simulink library "libraryMatlab"  (R2020b)
settings: Solver=VariableStepAuto  StartTime=0.0  StopTime=10.0  RelTol=1e-3
values from neighbouring files (symbols this model uses):
  a = 7271    [linearControlTuning.m]
  data = struct()    [config.m]
undefined symbols (not defined in the file or in its folder): SRP
libraries: simulink x2
settings Model: Creator=pacif  LastModifiedBy=pacif

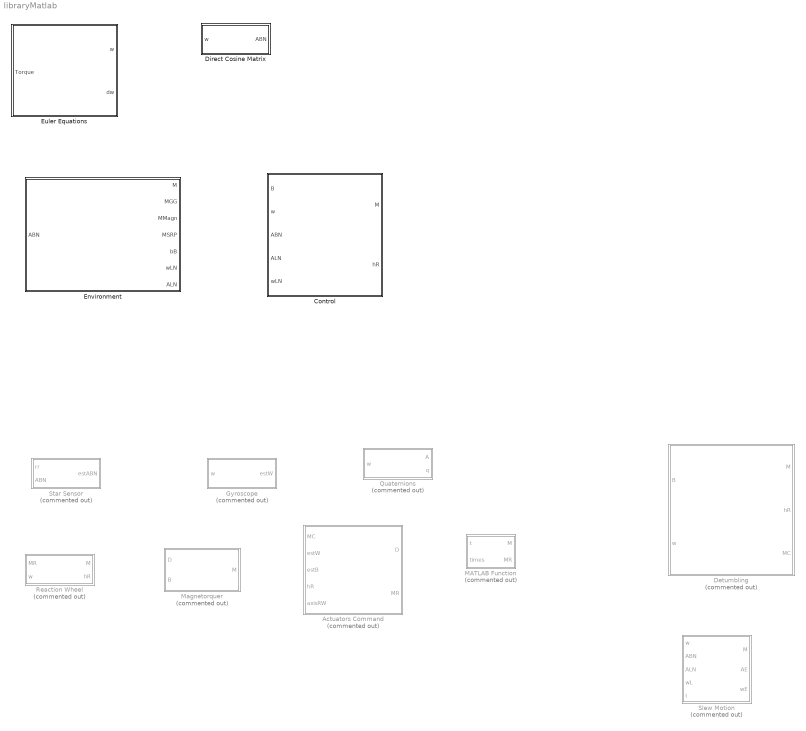
== system libraryMatlab ==
  Actuators Command : MATLAB Function  Commented=on  TreatAsAtomicUnit=on
  Control : Subsystem
  Detumbling : Subsystem  Commented=on
  Direct Cosine Matrix : Subsystem
  Environment : Subsystem
  Euler Equations : Subsystem
  Gyroscope : Subsystem  Commented=on
  MATLAB Function : MATLAB Function  Commented=on  TreatAsAtomicUnit=on
  Magnetorquer : MATLAB Function  Commented=on  TreatAsAtomicUnit=on
  Quaternions : Subsystem  Commented=on
  Reaction Wheel : Subsystem  Commented=on
  Slew Motion : MATLAB Function  Commented=on  TreatAsAtomicUnit=on
  Star Sensor : Subsystem  Commented=on

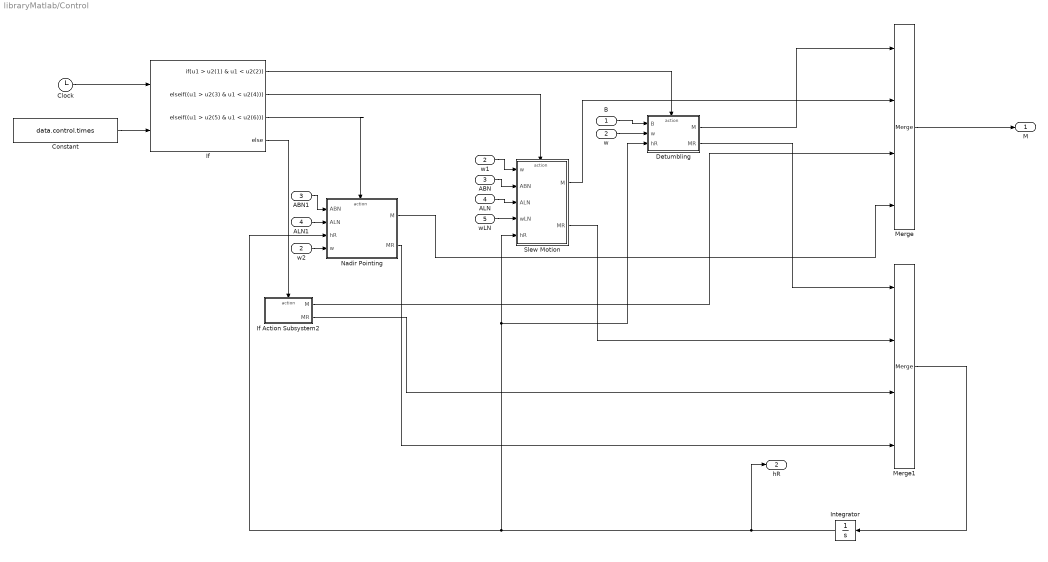
== system libraryMatlab/Control ==
  B : Inport
  w : Inport  Port=2
  ABN : Inport  Port=3
  ALN : Inport  Port=4
  wLN : Inport  Port=5
  ABN1 : InportShadow  Port=3
  ALN1 : InportShadow  Port=4
  Clock : Clock
  Constant : Constant  Value=data.control.times
  Detumbling : Subsystem  TreatAsAtomicUnit=on
  If : If  NumInputs=2  IfExpression=u1 > u2(1) & u1 < u2(2)  ElseIfExpressions=(u1 > u2(3) & u1 < u2(4)),(u1 > u2(5) & u1 < u2(6))
  If Action Subsystem2 : Subsystem  AncestorBlock=libraryMatlab/Control/Detumbling/If Action Subsystem2  TreatAsAtomicUnit=on
  Integrator : Integrator  InitialCondition=data.reactionWheel.h0
  Merge : Merge  Inputs=4
  Merge1 : Merge  Inputs=4
  Nadir Pointing : Subsystem  TreatAsAtomicUnit=on
  Slew Motion : Subsystem  TreatAsAtomicUnit=on
  w1 : InportShadow  Port=2
  w2 : InportShadow  Port=2
  M : Outport
  hR : Outport  Port=2
  wires:
  If/4 -> If Action Subsystem2/Action
  If/2 -> Slew Motion/Action
  If/1 -> Detumbling/Action
  Detumbling/1(M) -> Merge/1
  Slew Motion/1(M) -> Merge/2
  If Action Subsystem2/1(M) -> Merge/3
  Clock/1 -> If/1
  Constant/1 -> If/2
  B/1 -> Detumbling/1(B)
  w/1 -> Detumbling/2(w)
  w1/1 -> Slew Motion/1(w)
  ABN/1 -> Slew Motion/2(ABN)
  ALN/1 -> Slew Motion/3(ALN)
  wLN/1 -> Slew Motion/4(wLN)
  Merge/1 -> M/1
  Integrator/1 -> Nadir Pointing/3(hR), Detumbling/3(hR), Slew Motion/5(hR), hR/1
  Merge1/1 -> Integrator/1
  Detumbling/2(MR) -> Merge1/1
  Slew Motion/2(MR) -> Merge1/2
  If Action Subsystem2/2(MR) -> Merge1/3
  If/3 -> Nadir Pointing/Action
  Nadir Pointing/1(M) -> Merge/4
  ABN1/1 -> Nadir Pointing/1(ABN)
  ALN1/1 -> Nadir Pointing/2(ALN)
  Nadir Pointing/2(MR) -> Merge1/4
  w2/1 -> Nadir Pointing/4(w)

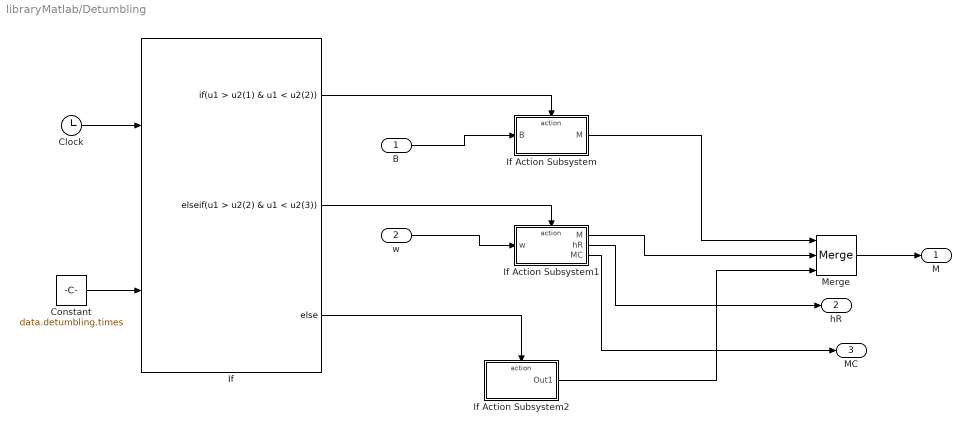
== system libraryMatlab/Detumbling ==
  B : Inport
  w : Inport  Port=2
  Clock : Clock
  Constant : Constant  Value=data.detumbling.times
  If : If  NumInputs=2  IfExpression=u1 > u2(1) & u1 < u2(2)  ElseIfExpressions=u1 > u2(2) & u1 < u2(3)
  If Action Subsystem : Subsystem  TreatAsAtomicUnit=on
  If Action Subsystem1 : Subsystem  TreatAsAtomicUnit=on
  If Action Subsystem2 : Subsystem  TreatAsAtomicUnit=on
  Merge : Merge  Inputs=3
  M : Outport
  hR : Outport  Port=2
  MC : Outport  Port=3
  wires:
  Clock/1 -> If/1
  If/1 -> If Action Subsystem/Action
  If/2 -> If Action Subsystem1/Action
  If/3 -> If Action Subsystem2/Action
  Merge/1 -> M/1
  If Action Subsystem2/1(Out1) -> Merge/3
  If Action Subsystem1/1(M) -> Merge/2
  If Action Subsystem/1(M) -> Merge/1
  B/1 -> If Action Subsystem/1(B)
  w/1 -> If Action Subsystem1/1(w)
  Constant/1 -> If/2
  If Action Subsystem1/2(hR) -> hR/1
  If Action Subsystem1/3(MC) -> MC/1

== system libraryMatlab/Direct Cosine Matrix ==
  w : Inport
  Integrator : Integrator  InitialCondition=data.ic.dcm
  MATLAB Function : MATLAB Function  TreatAsAtomicUnit=on
  MATLAB Function1 : MATLAB Function  TreatAsAtomicUnit=on
  ABN : Outport
  wires:
  w/1 -> MATLAB Function/2(w)
  MATLAB Function/1(dA) -> Integrator/1
  Integrator/1 -> MATLAB Function1/1(A0)
  MATLAB Function1/1(A) -> ABN/1, MATLAB Function/1(A)

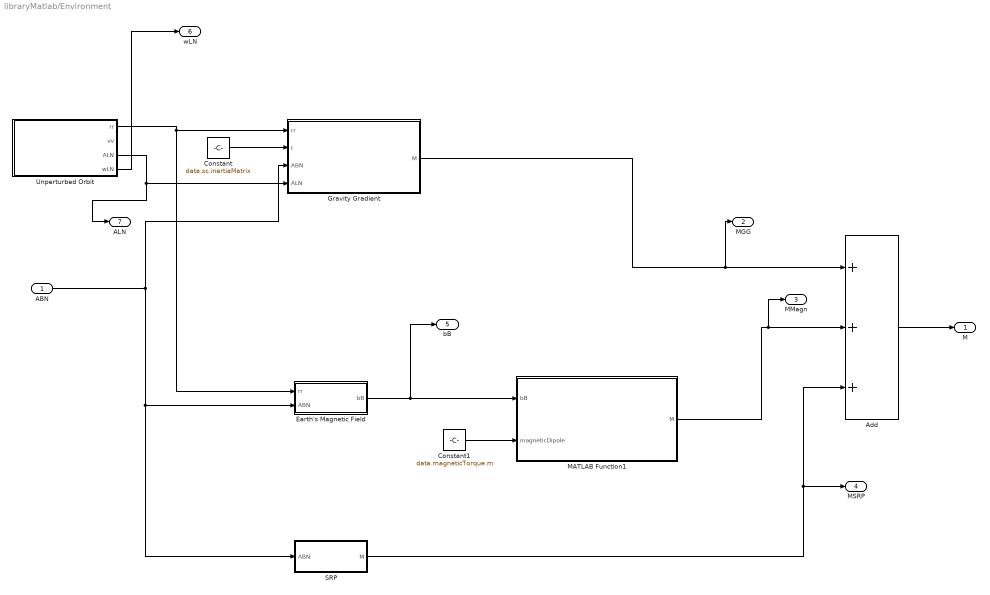
== system libraryMatlab/Environment ==
  ABN : Inport
  Add : Sum  Inputs=+++
  Constant : Constant  Value=data.sc.inertiaMatrix
  Constant1 : Constant  Value=data.magneticTorque.m
  Earth's Magnetic Field : Subsystem
  Gravity Gradient : MATLAB Function  TreatAsAtomicUnit=on
  MATLAB Function1 : MATLAB Function  TreatAsAtomicUnit=on
  SRP : Subsystem  AncestorBlock=a/SRP
  Unperturbed Orbit : Subsystem
  M : Outport
  MGG : Outport  Port=2
  MMagn : Outport  Port=3
  MSRP : Outport  Port=4
  bB : Outport  Port=5
  wLN : Outport  Port=6
  ALN : Outport  Port=7
  wires:
  Unperturbed Orbit/1(rr) -> Earth's Magnetic Field/1(rr), Gravity Gradient/1(rr)
  Unperturbed Orbit/3(ALN) -> ALN/1, Gravity Gradient/4(ALN)
  Constant/1 -> Gravity Gradient/2(I)
  Constant1/1 -> MATLAB Function1/2(magneticDipole)
  ABN/1 -> Gravity Gradient/3(ABN), Earth's Magnetic Field/2(ABN), SRP/1(ABN)
  MATLAB Function1/1(M) -> Add/2, MMagn/1
  Earth's Magnetic Field/1(bB) -> bB/1, MATLAB Function1/1(bB)
  Gravity Gradient/1(M) -> MGG/1, Add/1
  SRP/1(M) -> MSRP/1, Add/3
  Add/1 -> M/1
  Unperturbed Orbit/4(wLN) -> wLN/1

== system libraryMatlab/Euler Equations ==
  Torque : Inport
  Constant : Constant  Value=data.sc.inertiaMatrix
  Integrator : Integrator  InitialCondition=data.ic.w
  MATLAB Function : MATLAB Function  TreatAsAtomicUnit=on
  w : Outport
  dw : Outport  Port=2
  wires:
  Constant/1 -> MATLAB Function/3(I)
  Integrator/1 -> w/1, MATLAB Function/1(w)
  Torque/1 -> MATLAB Function/2(M)
  MATLAB Function/1(dw) -> dw/1, Integrator/1

== system libraryMatlab/Gyroscope ==
  w : Inport
  Add : Sum  Inputs=+++
  Band-Limited White Noise : simulink/Sources/Band-Limited White Noise  Cov=[1; 1; 1]  Ts=data.gyroscope.sampleTime  seed=[23341]
  Band-Limited White Noise1 : simulink/Sources/Band-Limited White Noise  Cov=[1; 1; 1]  Ts=data.gyroscope.sampleTime  seed=[23341]
  Gain : Gain  Gain=data.gyroscope.sigmaN
  Gain1 : Gain  Gain=data.gyroscope.sigmaB
  Integrator : Integrator  InitialCondition=[0;0;0]
  estW : Outport
  wires:
  Band-Limited White Noise/1 -> Gain/1
  Gain/1 -> Add/2  "n"
  Gain1/1 -> Integrator/1  "bDot"
  Integrator/1 -> Add/3  "b"
  w/1 -> Add/1
  Add/1 -> estW/1
  Band-Limited White Noise1/1 -> Gain1/1

== system libraryMatlab/Quaternions ==
  w : Inport
  Integrator : Integrator  InitialCondition=data.ic.quaternions
  MATLAB Function : MATLAB Function  TreatAsAtomicUnit=on
  MATLAB Function1 : MATLAB Function  TreatAsAtomicUnit=on
  MATLAB Function2 : MATLAB Function  TreatAsAtomicUnit=on
  A : Outport
  q : Outport  Port=2
  wires:
  w/1 -> MATLAB Function/2(w)
  MATLAB Function/1(dq) -> Integrator/1
  Integrator/1 -> MATLAB Function2/1(q0)
  MATLAB Function2/1(q) -> MATLAB Function/1(q), q/1, MATLAB Function1/1(q)
  MATLAB Function1/1(A) -> A/1

== system libraryMatlab/Reaction Wheel ==
  MR : Inport
  w : Inport  Port=2
  Constant : Constant  Value=data.reactionWheel.axes
  Integrator : Integrator
  MATLAB Function : MATLAB Function  TreatAsAtomicUnit=on
  M : Outport
  hR : Outport  Port=2
  wires:
  MR/1 -> MATLAB Function/2(MR), Integrator/1
  Integrator/1 -> hR/1, MATLAB Function/1(hR)  "hR"
  Constant/1 -> MATLAB Function/4(axesRW)
  w/1 -> MATLAB Function/3(w)
  MATLAB Function/1(M) -> M/1

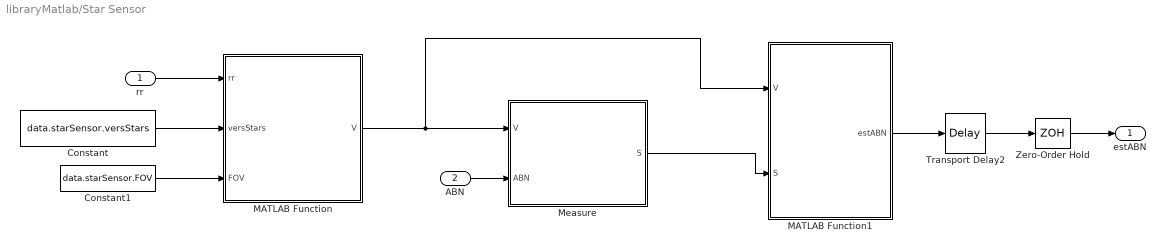
== system libraryMatlab/Star Sensor ==
  rr : Inport
  ABN : Inport  Port=2
  Constant : Constant  Value=data.starSensor.versStars
  Constant1 : Constant  Value=data.starSensor.FOV
  MATLAB Function : MATLAB Function  TreatAsAtomicUnit=on
  MATLAB Function1 : MATLAB Function  TreatAsAtomicUnit=on
  Measure : Subsystem
  Transport Delay2 : TransportDelay  DelayTime=data.starSensor.sampleTime
  Zero-Order Hold : ZeroOrderHold  SampleTime=data.starSensor.sampleTime
  estABN : Outport
  wires:
  Constant/1 -> MATLAB Function/2(versStars)
  Constant1/1 -> MATLAB Function/3(FOV)
  Measure/1(S) -> MATLAB Function1/2(S)
  ABN/1 -> Measure/2(ABN)
  Zero-Order Hold/1 -> estABN/1
  rr/1 -> MATLAB Function/1(rr)
  MATLAB Function/1(V) -> MATLAB Function1/1(V), Measure/1(V)
  MATLAB Function1/1(estABN) -> Transport Delay2/1
  Transport Delay2/1 -> Zero-Order Hold/1

== system libraryMatlab/Control/Detumbling ==
  B : Inport
  w : Inport  Port=2
  hR : Inport  Port=3
  Action Port : ActionPort  ActionPortLabel=if(u1 > u2(1) & u1 < u2(2))
  Detumbling : Subsystem  AncestorBlock=libraryMatlab/Detumbling
  M : Outport
  MR : Outport  Port=2
  wires:
  Detumbling/1(M) -> M/1
  B/1 -> Detumbling/1(B)
  w/1 -> Detumbling/2(w)
  Detumbling/2(MR) -> MR/1
  hR/1 -> Detumbling/3(hR)

== system libraryMatlab/Control/If Action Subsystem2 ==
  Action Port : ActionPort  ActionPortLabel=else
  Constant : Constant  Value=[0;0;0]
  Constant1 : Constant  Value=0*data.reactionWheel.h0  VectorParams1D=off
  M : Outport
  MR : Outport  Port=2
  wires:
  Constant/1 -> M/1
  Constant1/1 -> MR/1

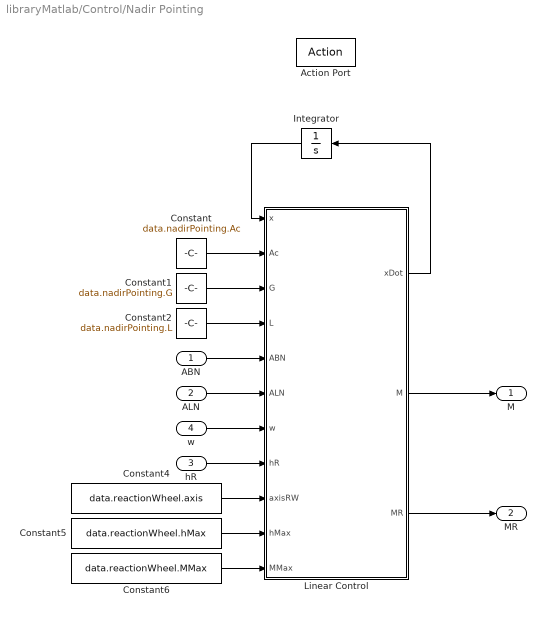
== system libraryMatlab/Control/Nadir Pointing ==
  ABN : Inport
  ALN : Inport  Port=2
  hR : Inport  Port=3
  w : Inport  Port=4
  Action Port : ActionPort  ActionPortLabel=elseif((u1 > u2(5) & u1 < u2(6)))
  Constant : Constant  Value=data.nadirPointing.Ac
  Constant1 : Constant  Value=data.nadirPointing.G
  Constant2 : Constant  Value=data.nadirPointing.L
  Constant4 : Constant  Value=data.reactionWheel.axis
  Constant5 : Constant  Value=data.reactionWheel.hMax
  Constant6 : Constant  Value=data.reactionWheel.MMax
  Integrator : Integrator  InitialCondition=zeros(6,1)
  Linear Control : MATLAB Function  TreatAsAtomicUnit=on
  M : Outport
  MR : Outport  Port=2
  wires:
  ALN/1 -> Linear Control/6(ALN)
  ABN/1 -> Linear Control/5(ABN)
  Linear Control/2(M) -> M/1
  Linear Control/1(xDot) -> Integrator/1
  Integrator/1 -> Linear Control/1(x)
  Constant/1 -> Linear Control/2(Ac)
  Constant2/1 -> Linear Control/4(L)
  Constant1/1 -> Linear Control/3(G)
  Constant4/1 -> Linear Control/9(axisRW)
  Constant5/1 -> Linear Control/10(hMax)
  Constant6/1 -> Linear Control/11(MMax)
  hR/1 -> Linear Control/8(hR)
  Linear Control/3(MR) -> MR/1
  w/1 -> Linear Control/7(w)

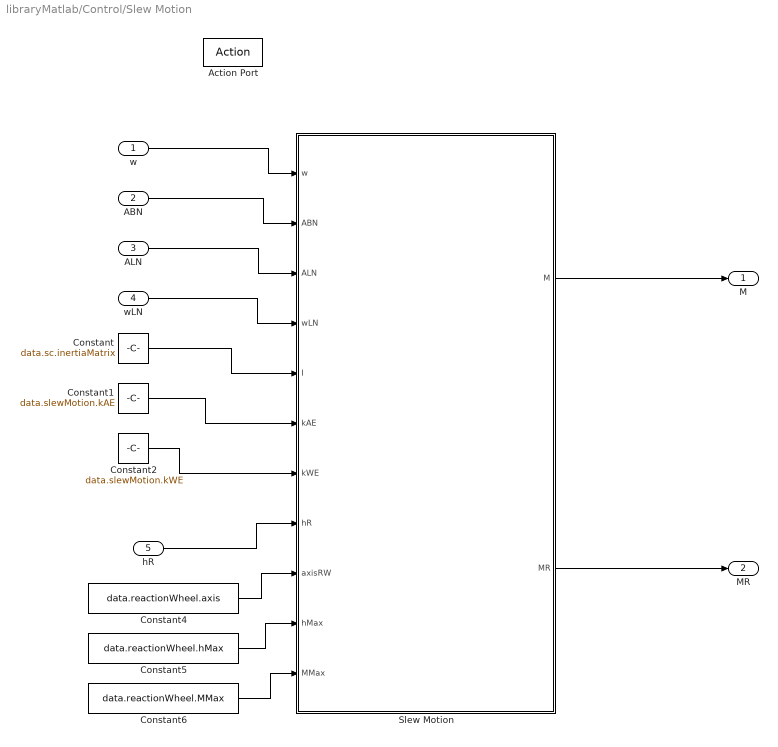
== system libraryMatlab/Control/Slew Motion ==
  w : Inport
  ABN : Inport  Port=2
  ALN : Inport  Port=3
  wLN : Inport  Port=4
  hR : Inport  Port=5
  Action Port : ActionPort  ActionPortLabel=elseif(u1 > u2(3) & u1 < u2(4))
  Constant : Constant  Value=data.sc.inertiaMatrix
  Constant1 : Constant  Value=data.slewMotion.kAE
  Constant2 : Constant  Value=data.slewMotion.kWE
  Constant4 : Constant  Value=data.reactionWheel.axis
  Constant5 : Constant  Value=data.reactionWheel.hMax
  Constant6 : Constant  Value=data.reactionWheel.MMax
  Slew Motion : MATLAB Function  TreatAsAtomicUnit=on
  M : Outport
  MR : Outport  Port=2
  wires:
  Slew Motion/1(M) -> M/1
  w/1 -> Slew Motion/1(w)
  ABN/1 -> Slew Motion/2(ABN)
  ALN/1 -> Slew Motion/3(ALN)
  wLN/1 -> Slew Motion/4(wLN)
  Constant/1 -> Slew Motion/5(I)
  Constant1/1 -> Slew Motion/6(kAE)
  Constant2/1 -> Slew Motion/7(kWE)
  Slew Motion/2(MR) -> MR/1
  hR/1 -> Slew Motion/8(hR)
  Constant5/1 -> Slew Motion/10(hMax)
  Constant4/1 -> Slew Motion/9(axisRW)
  Constant6/1 -> Slew Motion/11(MMax)

== system libraryMatlab/Detumbling/If Action Subsystem ==
  B : Inport
  Action Port : ActionPort  ActionPortLabel=if(u1 > u2(1) & u1 < u2(2))
  Constant : Constant  Value=data.magnetorquer.m0
  Derivative : Derivative  CoefficientInTFapproximation=0
  Spin Rate Damping : MATLAB Function  TreatAsAtomicUnit=on
  M : Outport
  wires:
  Constant/1 -> Spin Rate Damping/1(m0)
  B/1 -> Spin Rate Damping/2(B), Derivative/1
  Spin Rate Damping/1(M) -> M/1
  Derivative/1 -> Spin Rate Damping/3(BDot)

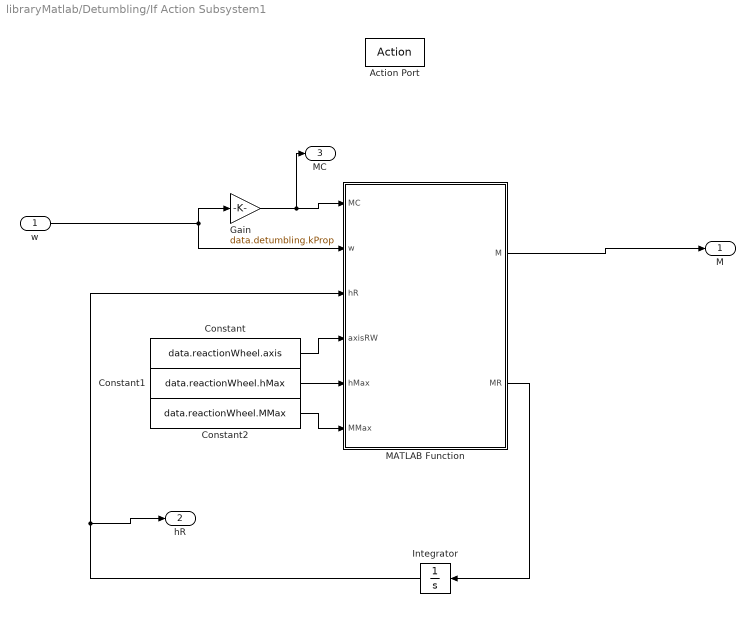
== system libraryMatlab/Detumbling/If Action Subsystem1 ==
  w : Inport
  Action Port : ActionPort  ActionPortLabel=elseif(u1 > u2(2) & u1 < u2(3))
  Constant : Constant  Value=data.reactionWheel.axis
  Constant1 : Constant  Value=data.reactionWheel.hMax
  Constant2 : Constant  Value=data.reactionWheel.MMax
  Gain : Gain  Gain=data.detumbling.kProp
  Integrator : Integrator  InitialCondition=data.reactionWheel.h0
  MATLAB Function : MATLAB Function  TreatAsAtomicUnit=on
  M : Outport
  hR : Outport  Port=2
  MC : Outport  Port=3
  wires:
  w/1 -> Gain/1, MATLAB Function/2(w)
  Gain/1 -> MC/1, MATLAB Function/1(MC)
  MATLAB Function/2(MR) -> Integrator/1
  MATLAB Function/1(M) -> M/1
  Constant/1 -> MATLAB Function/4(axisRW)
  Constant1/1 -> MATLAB Function/5(hMax)
  Constant2/1 -> MATLAB Function/6(MMax)
  Integrator/1 -> hR/1, MATLAB Function/3(hR)

== system libraryMatlab/Detumbling/If Action Subsystem2 ==
  Action Port : ActionPort  ActionPortLabel=else
  Constant : Constant  Value=[0;0;0]
  Out1 : Outport
  wires:
  Constant/1 -> Out1/1

== system libraryMatlab/Environment/Earth's Magnetic Field ==
  rr : Inport
  ABN : Inport  Port=2
  Clock : Clock
  Earth's Magnetic Field : MATLAB Function  TreatAsAtomicUnit=on
  bB : Outport
  wires:
  Earth's Magnetic Field/1(bB) -> bB/1
  rr/1 -> Earth's Magnetic Field/2(rr)
  ABN/1 -> Earth's Magnetic Field/3(ABN)
  Clock/1 -> Earth's Magnetic Field/1(t)

== system libraryMatlab/Environment/SRP ==
  ABN : Inport
  Clock : Clock
  Constant : Constant  Value=data.SRP.rhoS
  Constant1 : Constant  Value=data.SRP.rhoD
  Constant2 : Constant  Value=data.SRP.NBMat
  Constant3 : Constant  Value=data.SRP.rSurf
  Constant4 : Constant  Value=data.SRP.aSurf
  MATLAB Function : MATLAB Function  TreatAsAtomicUnit=on
  M : Outport
  wires:
  Constant4/1 -> MATLAB Function/7(aSurf)
  Constant3/1 -> MATLAB Function/6(rSurf)
  Constant2/1 -> MATLAB Function/5(NBMat)
  Constant1/1 -> MATLAB Function/4(rhoD)
  Constant/1 -> MATLAB Function/3(rhoS)
  Clock/1 -> MATLAB Function/1(t)
  MATLAB Function/1(M) -> M/1
  ABN/1 -> MATLAB Function/2(ABN)

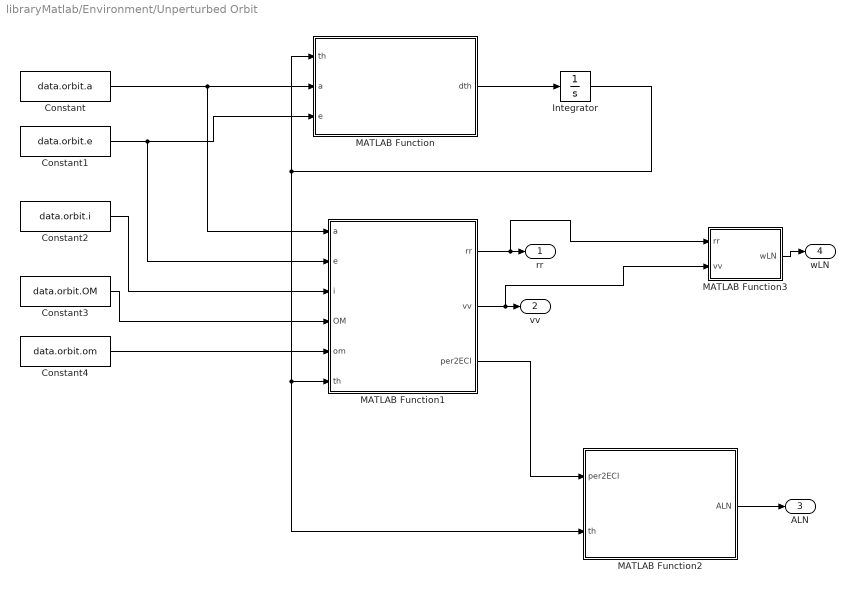
== system libraryMatlab/Environment/Unperturbed Orbit ==
  Constant : Constant  Value=data.orbit.a
  Constant1 : Constant  Value=data.orbit.e
  Constant2 : Constant  Value=data.orbit.i
  Constant3 : Constant  Value=data.orbit.OM
  Constant4 : Constant  Value=data.orbit.om
  Integrator : Integrator  InitialCondition=data.ic.th
  MATLAB Function : MATLAB Function  TreatAsAtomicUnit=on
  MATLAB Function1 : MATLAB Function  TreatAsAtomicUnit=on
  MATLAB Function2 : MATLAB Function  TreatAsAtomicUnit=on
  MATLAB Function3 : MATLAB Function  TreatAsAtomicUnit=on
  rr : Outport
  vv : Outport  Port=2
  ALN : Outport  Port=3
  wLN : Outport  Port=4
  wires:
  Constant/1 -> MATLAB Function1/1(a), MATLAB Function/2(a)
  Constant1/1 -> MATLAB Function1/2(e), MATLAB Function/3(e)
  MATLAB Function/1(dth) -> Integrator/1
  Integrator/1 -> MATLAB Function2/2(th), MATLAB Function1/6(th), MATLAB Function/1(th)
  Constant2/1 -> MATLAB Function1/3(i)
  Constant3/1 -> MATLAB Function1/4(OM)
  Constant4/1 -> MATLAB Function1/5(om)
  MATLAB Function1/1(rr) -> MATLAB Function3/1(rr), rr/1
  MATLAB Function1/2(vv) -> MATLAB Function3/2(vv), vv/1
  MATLAB Function1/3(per2ECI) -> MATLAB Function2/1(per2ECI)
  MATLAB Function2/1(ALN) -> ALN/1
  MATLAB Function3/1(wLN) -> wLN/1

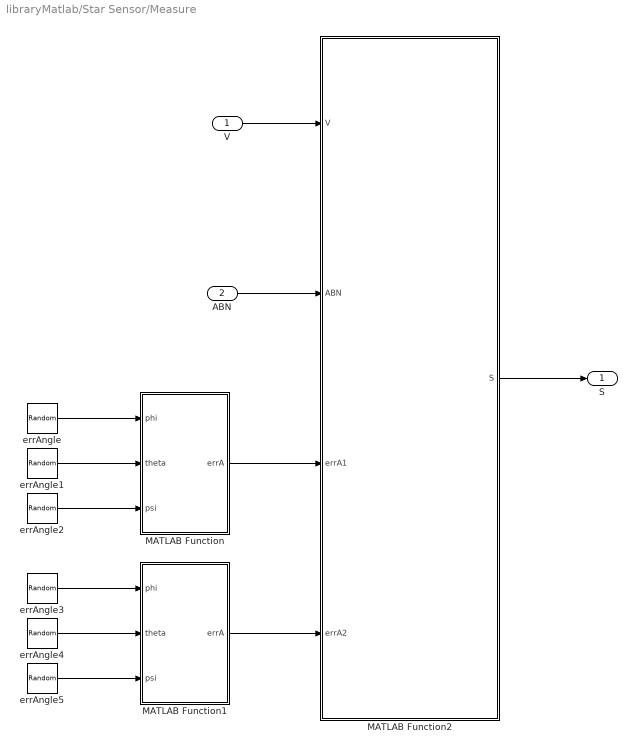
== system libraryMatlab/Star Sensor/Measure ==
  V : Inport
  ABN : Inport  Port=2
  MATLAB Function : MATLAB Function  TreatAsAtomicUnit=on
  MATLAB Function1 : MATLAB Function  TreatAsAtomicUnit=on
  MATLAB Function2 : MATLAB Function  TreatAsAtomicUnit=on
  errAngle{,1..5} (6 alike) : RandomNumber  Variance=data.starSensor.variance  SampleTime=data.starSensor.sampleTime
  S : Outport
  wires:
  errAngle/1 -> MATLAB Function/1(phi)
  errAngle1/1 -> MATLAB Function/2(theta)
  errAngle2/1 -> MATLAB Function/3(psi)
  errAngle5/1 -> MATLAB Function1/3(psi)
  errAngle4/1 -> MATLAB Function1/2(theta)
  errAngle3/1 -> MATLAB Function1/1(phi)
  MATLAB Function/1(errA) -> MATLAB Function2/3(errA1)
  MATLAB Function1/1(errA) -> MATLAB Function2/4(errA2)
  MATLAB Function2/1(S) -> S/1
  V/1 -> MATLAB Function2/1(V)
  ABN/1 -> MATLAB Function2/2(ABN)

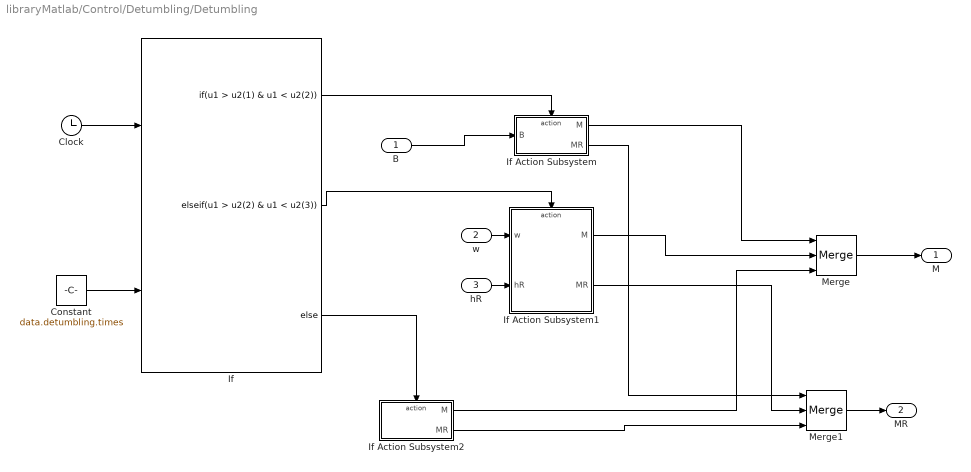
== system libraryMatlab/Control/Detumbling/Detumbling ==
  B : Inport
  w : Inport  Port=2
  hR : Inport  Port=3
  Clock : Clock
  Constant : Constant  Value=data.detumbling.times
  If : If  NumInputs=2  IfExpression=u1 > u2(1) & u1 < u2(2)  ElseIfExpressions=u1 > u2(2) & u1 < u2(3)
  If Action Subsystem : Subsystem  TreatAsAtomicUnit=on
  If Action Subsystem1 : Subsystem  TreatAsAtomicUnit=on
  If Action Subsystem2 : Subsystem  TreatAsAtomicUnit=on
  Merge : Merge  Inputs=3
  Merge1 : Merge  Inputs=3
  M : Outport
  MR : Outport  Port=2
  wires:
  Constant/1 -> If/2
  w/1 -> If Action Subsystem1/1(w)
  B/1 -> If Action Subsystem/1(B)
  If Action Subsystem/1(M) -> Merge/1
  If Action Subsystem1/1(M) -> Merge/2
  If Action Subsystem2/1(M) -> Merge/3
  Merge/1 -> M/1
  If/3 -> If Action Subsystem2/Action
  If/2 -> If Action Subsystem1/Action
  If/1 -> If Action Subsystem/Action
  Clock/1 -> If/1
  If Action Subsystem1/2(MR) -> Merge1/2
  hR/1 -> If Action Subsystem1/2(hR)
  Merge1/1 -> MR/1
  If Action Subsystem2/2(MR) -> Merge1/3
  If Action Subsystem/2(MR) -> Merge1/1

== system libraryMatlab/Control/Detumbling/Detumbling/If Action Subsystem ==
  B : Inport
  Action Port : ActionPort
  Constant : Constant  Value=data.magnetorquer.m0
  Constant1 : Constant  Value=0*data.reactionWheel.h0  VectorParams1D=off
  Derivative : Derivative  CoefficientInTFapproximation=0
  Spin Rate Damping : MATLAB Function  TreatAsAtomicUnit=on
  M : Outport
  MR : Outport  Port=2
  wires:
  Derivative/1 -> Spin Rate Damping/3(BDot)
  Spin Rate Damping/1(M) -> M/1
  B/1 -> Derivative/1, Spin Rate Damping/2(B)
  Constant/1 -> Spin Rate Damping/1(m0)
  Constant1/1 -> MR/1

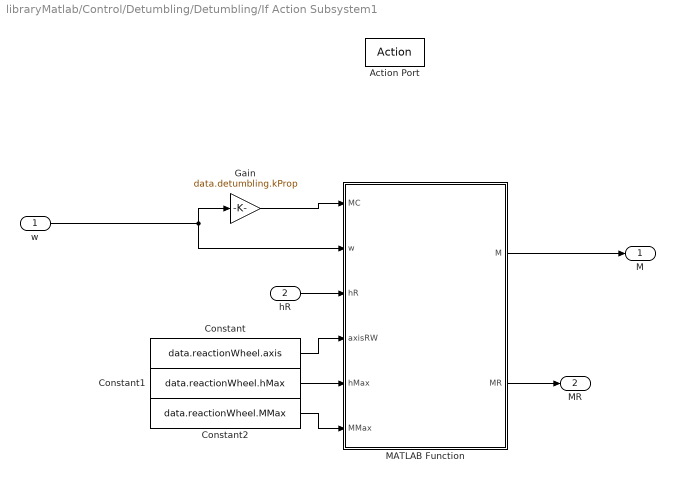
== system libraryMatlab/Control/Detumbling/Detumbling/If Action Subsystem1 ==
  w : Inport
  hR : Inport  Port=2
  Action Port : ActionPort
  Constant : Constant  Value=data.reactionWheel.axis
  Constant1 : Constant  Value=data.reactionWheel.hMax
  Constant2 : Constant  Value=data.reactionWheel.MMax
  Gain : Gain  Gain=data.detumbling.kProp
  MATLAB Function : MATLAB Function  TreatAsAtomicUnit=on
  M : Outport
  MR : Outport  Port=2
  wires:
  Constant2/1 -> MATLAB Function/6(MMax)
  Constant1/1 -> MATLAB Function/5(hMax)
  Constant/1 -> MATLAB Function/4(axisRW)
  MATLAB Function/1(M) -> M/1
  MATLAB Function/2(MR) -> MR/1
  Gain/1 -> MATLAB Function/1(MC)
  w/1 -> MATLAB Function/2(w), Gain/1
  hR/1 -> MATLAB Function/3(hR)

== system libraryMatlab/Control/Detumbling/Detumbling/If Action Subsystem2 ==
  Action Port : ActionPort
  Constant : Constant  Value=[0;0;0]
  Constant1 : Constant  Value=0*data.reactionWheel.h0  VectorParams1D=off
  M : Outport
  MR : Outport  Port=2
  wires:
  Constant/1 -> M/1
  Constant1/1 -> MR/1

== matlab function libraryMatlab/Environment/Unperturbed Orbit/MATLAB Function2 ==
  data: per2ECI input; ALN output; th input
function ALN = computeALN(per2ECI,th)

ECI2per = per2ECI';

per2L = [cos(th)  sin(th)  0;
        -sin(th)  cos(th)  0;
            0        0     1];
        
ALN = per2L*ECI2per;

end

== matlab function libraryMatlab/Environment/MATLAB Function1 ==
  data: bB input; M output; magneticDipole input
function M = magneticTorque(bB,magneticDipole)

M = cross(magneticDipole,bB); 

end

== matlab function libraryMatlab/Environment/SRP/MATLAB Function ==
  data: t input; ABN input; M output; rhoS input; rhoD input; NBMat input; rSurf input; aSurf input
function M = SRP(t,ABN,rhoS,rhoD,NBMat,rSurf,aSurf)

% Constants:
Fe = 2081.4; c = 3e8; P = Fe/c;

N_SUN = 2*pi/365/24/3600; OBL = 23.45*pi/180;
R_SUN = 1.496e8;

SN = R_SUN*[cos(N_SUN*t); 
    sin(N_SUN*t)*cos(OBL);
    sin(N_SUN*t)*sin(OBL)];
SN = SN/norm(SN);

SB = ABN*SN;

nSurf = size(NBMat,2);

M = [0; 0; 0];

for i = 1:nSurf
    
    NBi = NBMat(:,i); ri = rSurf(:,i); Ai = aSurf(i);
    rhoSi = rhoS(i); rhoDi = rhoD(i);
    
    Ki = dot(SB,NBi); 
    
    if Ki > 0
        
        Fi = -P*Ai*Ki*((1-rhoSi)*SB +...
            (2*rhoSi*Ki + 2/3*rhoDi)*NBi);
        
        M = M + cross(ri,Fi);
        
    end
    
end

end

== matlab function libraryMatlab/Star Sensor/MATLAB Function ==
  data: rr input; V output; versStars input; FOV input
function V = starCatalog(rr,versStars,FOV)

rrVers = rr/norm(rr);

% Search on star catalogue:

angles = acos(versStars*rrVers);

anglesInFOV = angles < FOV;

starsInFOV = versStars(anglesInFOV,:);

nMeasures = 2;

V = starsInFOV(1:nMeasures,:)';

== matlab function libraryMatlab/Star Sensor/MATLAB Function1 ==
  data: V input; estABN output; S input
function estABN = attitudeEstimation(V,S)

p = S(:,1); q = S(:,2); a = V(:,1); b = V(:,2);

m1 = p; 
m2 = cross(p,q); m2 = m2/norm(m2);
m3 = cross(p,m2);

n1 = a; 
n2 = cross(a,b); n2 = n2/norm(n2);
n3 = cross(a,n2);

M = [m1, m2, m3]; N = [n1, n2, n3];

estABN = M*N';

== matlab function libraryMatlab/Star Sensor/Measure/MATLAB Function ==
  data: phi input; errA output; theta input; psi input
function errA = errorRotation(phi,theta,psi)

errA = [ cos(psi)*cos(theta), cos(phi)*sin(psi) + cos(psi)*sin(phi)*sin(theta), sin(phi)*sin(psi) - cos(phi)*cos(psi)*sin(theta)
-cos(theta)*sin(psi), cos(phi)*cos(psi) - sin(phi)*sin(psi)*sin(theta), cos(psi)*sin(phi) + cos(phi)*sin(psi)*sin(theta)
          sin(theta),                             -cos(theta)*sin(phi),                              cos(phi)*cos(theta)];

== matlab function libraryMatlab/Star Sensor/Measure/MATLAB Function1 ==
  data: phi input; errA output; theta input; psi input
function errA = errorRotation(phi,theta,psi)

errA = [ cos(psi)*cos(theta), cos(phi)*sin(psi) + cos(psi)*sin(phi)*sin(theta), sin(phi)*sin(psi) - cos(phi)*cos(psi)*sin(theta)
-cos(theta)*sin(psi), cos(phi)*cos(psi) - sin(phi)*sin(psi)*sin(theta), cos(psi)*sin(phi) + cos(phi)*sin(psi)*sin(theta)
          sin(theta),                             -cos(theta)*sin(phi),                              cos(phi)*cos(theta)];

== matlab function libraryMatlab/Star Sensor/Measure/MATLAB Function2 ==
  data: V input; S output; ABN input; errA1 input; errA2 input
function S = measure(V,ABN,errA1,errA2)

r1 = V(:,1); r2 = V(:,2);

s1 = errA1*ABN*r1; s2 = errA2*ABN*r2;

S = [s1, s2];

== matlab function libraryMatlab/Reaction Wheel/MATLAB Function ==
  data: hR input; M output; MR input; w input; axesRW input
function M = reactionWheel(hR,MR,w,axesRW)

M = -cross(w,axesRW*hR) - axesRW*MR;

end

== matlab function libraryMatlab/Magnetorquer ==
  data: D input; M output; B input
function M = fun(D,B)

M = cross(D,B);

end

== matlab function libraryMatlab/Actuators Command ==
  data: MC input; D output; estW input; estB input; hR input; axisRW input; MR output
function [D,MR] = fun(MC, estW, estB, hR, axisRW)

M = MC + cross(estW,hR*axisRW);

Bx = estB(1); By = estB(2); Bz = estB(3);

Dx = M(2)/Bz; Dy = -M(1)/Bz;

MR = -M(3) + By*Dx - Bx*Dy;

D = [Dx; Dy; 0]; 

end

== matlab function libraryMatlab/Environment/Earth's Magnetic Field/Earth's Magnetic Field ==
  data: t input; bB output; rr input; ABN input
function bB = fcn(t,rr,ABN)

% Coefficients for 2020:
g10 = -29615e-9; g11 = -1728e-9; h11 = 5186e-9;
H0 = sqrt(g10^2 + g11^2 + h11^2);

OBL = 11.5*pi/180;
W_EARTH = (2*pi + 2*pi/365.26)/24/3600;
R_EARTH = 6371.0088;

mVers = [sin(OBL)*cos(W_EARTH*t);
        sin(OBL)*sin(W_EARTH*t);
        cos(OBL)];

rVers = rr/norm(rr);
rNorm = norm(rr);

bN = R_EARTH^3/rNorm^3*H0*(3*dot(mVers,rVers)*rVers - mVers);

bB = ABN*bN;

end

== matlab function libraryMatlab/Direct Cosine Matrix/MATLAB Function ==
  data: A input; dA output; w input
function dA = derivativeDCM(A,w)

M = [ 0 -w(3) w(2); 
    w(3) 0 -w(1);
    -w(2) w(1) 0];

dA = -M*A;


end

== matlab function libraryMatlab/Detumbling/If Action Subsystem1/MATLAB Function ==
  data: MC input; M output; w input; hR input; axisRW input; hMax input; MMax input; MR output
function [M,MR] = fcn(MC, w, hR, axisRW, hMax, MMax)

MR = -axisRW\(MC + cross(w,axisRW*hR));
% RW saturation:
for i = 1:length(MR)
    
    if abs(MR(i)) > MMax; MR(i) = sign(MR(i))*MMax; end
    if hR(i) >= hMax && MR(i) > 0, MR(i) = 0; end
    if hR(i) <= -hMax && MR(i) < 0, MR(i) = 0; end
    
end

M = -cross(w,axisRW*hR) - axisRW*MR;

end

== matlab function libraryMatlab/MATLAB Function ==
  data: t input; M output; times input; MR output
function [M,MR] = fcn(t,times)

M = [0;0;0]; MR = 0;

if t > times(1) && t < times(2)
    
    
    
    
    
    
elseif t > times(2) && t < times(3)
    
end

== matlab function libraryMatlab/Detumbling/If Action Subsystem/Spin Rate Damping ==
  data: m0 input; M output; B input; BDot input
function M = fcn(m0,B,BDot)

M = - cross(m0*sign(BDot),B);

== matlab function libraryMatlab/Environment/Unperturbed Orbit/MATLAB Function3 ==
  data: rr input; wLN output; vv input
function wLN = fcn(rr,vv)

MU = 398600;

n = sqrt(MU/(norm(rr)^3));

h = cross(rr,vv); 

wLN = h/norm(h)*n;

== matlab function libraryMatlab/Slew Motion ==
  data: w input; M output; ABN input; ALN input; wL input; I input; AE output; wE output
function [M,AE,wE] = fcn(w,ABN,ALN,wL,I)

wL = ABN*wL;

k1 = 1e-3; k2 = 1e-3;

AE = ABN*ALN'; 

wE = w - AE*wL;

AEV = [AE(2,3) - AE(3,2);
       AE(3,1) - AE(1,3);
       AE(1,2) - AE(2,1)];

M = -k1*wE - k2*AEV + cross(w,I*w) - I*cross(wE,AE*wL);

wE = w - wL;

== matlab function libraryMatlab/Control/Slew Motion/Slew Motion ==
  data: w input; M output; ABN input; ALN input; wLN input; I input; kAE input; kWE input; hR input; axisRW input; hMax input; MMax input; MR output
function [M,MR]  = fcn(w,ABN,ALN,wLN,I,kAE,kWE,hR, axisRW, hMax, MMax)

Ad = ALN;

wd = Ad*wLN;

AE = ABN*Ad'; 

wE = w - AE*wd;

AEV = [AE(2,3) - AE(3,2);
       AE(3,1) - AE(1,3);
       AE(1,2) - AE(2,1)];

MC = -kWE*wE - kAE*AEV + cross(w,I*w) - I*cross(wE,AE*wd);

MR = -axisRW\(MC + cross(w,axisRW*hR));
% RW saturation:
for i = 1:length(MR)
    
    if abs(MR(i)) > MMax; MR(i) = sign(MR(i))*MMax; end
    if hR(i) >= hMax && MR(i) > 0, MR(i) = 0; end
    if hR(i) <= -hMax && MR(i) < 0, MR(i) = 0; end
    
end

M = -cross(w,axisRW*hR) - axisRW*MR;

== matlab function libraryMatlab/Control/Detumbling/Detumbling/If Action Subsystem/Spin Rate Damping ==
  data: m0 input; M output; B input; BDot input
function M = fcn(m0,B,BDot)

M = - cross(m0*sign(BDot),B);

== matlab function libraryMatlab/Euler Equations/MATLAB Function ==
  data: w input; dw output; M input; I input
function dw = eulerEquations(w,M,I)

dw = I\(cross(I*w,w) + M);

end

== matlab function libraryMatlab/Control/Detumbling/Detumbling/If Action Subsystem1/MATLAB Function ==
  data: MC input; M output; w input; hR input; axisRW input; hMax input; MMax input; MR output
function [M,MR] = fcn(MC, w, hR, axisRW, hMax, MMax)

MR = -axisRW\(MC + cross(w,axisRW*hR));
% RW saturation:
for i = 1:length(MR)
    
    if abs(MR(i)) > MMax; MR(i) = sign(MR(i))*MMax; end
    if hR(i) >= hMax && MR(i) > 0, MR(i) = 0; end
    if hR(i) <= -hMax && MR(i) < 0, MR(i) = 0; end
    
end

M = -cross(w,axisRW*hR) - axisRW*MR;

end

== matlab function libraryMatlab/Control/Nadir Pointing/Linear Control ==
  data: x input; xDot output; Ac input; G input; L input; ABN input; ALN input; w input; M output; hR input; axisRW input; hMax input; MMax input; MR output
function [xDot,M,MR] = fcn(x,Ac,G,L,ABN,ALN,w, hR, axisRW, hMax, MMax)

ABL = ABN*ALN';

y = [0;0;0];

y(1) = 0.5*(ABL(2,3) - ABL(3,2));
y(2) = 0.5*(ABL(3,1) - ABL(1,3));
y(3) = 0.5*(ABL(1,2) - ABL(2,1));

xDot = Ac*x + L*y;

MC = -G*x;

wEst = x(4:6) + [0; 0; sqrt(398600/7271^3)];

MR = -axisRW\(MC + cross(wEst,axisRW*hR));
% RW saturation:
for i = 1:length(MR)
    
    if abs(MR(i)) > MMax; MR(i) = sign(MR(i))*MMax; end
    if hR(i) >= hMax && MR(i) > 0, MR(i) = 0; end
    if hR(i) <= -hMax && MR(i) < 0, MR(i) = 0; end
    
end

M = -cross(w,axisRW*hR) - axisRW*MR;

== matlab function libraryMatlab/Direct Cosine Matrix/MATLAB Function1 ==
  data: A0 input; A output
function A = orthonormalizeA(A0)

A = A0*3/2 - A0*(A0')*A0/2;

end

== matlab function libraryMatlab/Quaternions/MATLAB Function ==
  data: q input; dq output; w input
function dq = derivativeQuaternions(q,w)

w1 = w(1); w2 = w(2); w3 = w(3);

M = [0 w3 -w2 w1; 
    -w3 0 w1 w2;
    w2 -w1 0 w3;
    -w1 -w2 -w3 0];

dq = 0.5*M*q;

end

== matlab function libraryMatlab/Quaternions/MATLAB Function1 ==
  data: q input; A output
function A = quatToDCM(q)

q1 = q(1); q2 = q(2); q3 = q(3); q4 = q(4);

A = [ q1^2-q2^2-q3^2+q4^2    2*(q1*q2+q3*q4)        2*(q1*q3-q2*q4);
    2*(q1*q2-q3*q4)          -q1^2+q2^2-q3^2+q4^2   2*(q2*q3+q1*q4);
    2*(q1*q3+q2*q4)          2*(q2*q3-q1*q4)        -q1^2-q2^2+q3^2+q4^2];

end

== matlab function libraryMatlab/Quaternions/MATLAB Function2 ==
  data: q0 input; q output
function q = normalizeQuat(q0)

q = q0/norm(q0);
q = q0;

end

== matlab function libraryMatlab/Environment/Gravity Gradient ==
  data: rr input; M output; I input; ABN input; ALN input
function M = fun(rr,I,ABN,ALN)

MU = 398600;

Ix = I(1,1); Iy = I(2,2); Iz = I(3,3);

R = norm(rr);

ABL = ABN*ALN';

c = ABL*[1;0;0];

K = 3*MU/R^3;

M = K*[ (Iz - Iy)*c(3)*c(2);
        (Ix - Iz)*c(1)*c(3);
        (Iy - Ix)*c(2)*c(1)  ];
    
end

== matlab function libraryMatlab/Environment/Unperturbed Orbit/MATLAB Function ==
  data: th input; dth output; a input; e input
function dth = thetaDot(th, a, e)

MU = 398600;

n = sqrt(MU/a^3);

dth = n*(1 + e*cos(th))^2/(1 - e^2)^(3/2);

end

== matlab function libraryMatlab/Environment/Unperturbed Orbit/MATLAB Function1 ==
  data: a input; rr output; e input; i input; OM input; om input; th input; vv output; per2ECI output
function [rr,vv,per2ECI] = kep2car(a,e,i,OM,om,th)

MU = 398600;

p = a*(1-e^2);
r = p/(1+e*cos(th));

rr = r*[cos(th);sin(th);0];
vv = sqrt(MU/p)*[-sin(th);e+cos(th);0];

ROM = [ cos(OM) sin(OM) 0; -sin(OM) cos(OM) 0; 0 0 1];
Ri = [ 1 0 0; 0 cos(i) sin(i); 0 -sin(i) cos(i)];
Rom = [ cos(om) sin(om) 0; -sin(om) cos(om) 0; 0 0 1];

per2ECI = (Rom*Ri*ROM)';

rr = per2ECI*rr;
vv = per2ECI*vv;

end
